simulink model "TP2"  (R2020a)
settings: Solver=VariableStepAuto  StartTime=0.0  StopTime=10.0  RelTol=1e-3
libraries: dspsigops x2, commutil2 x2, commrandsrc3 x1
settings Model: Creator=acer  LastModifiedBy=acer

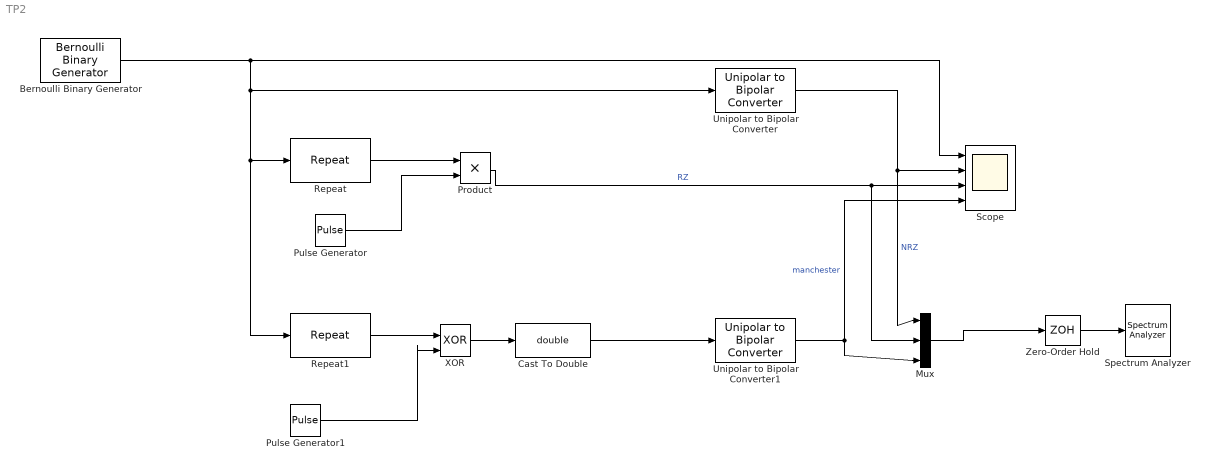
== system TP2 ==
  Bernoulli Binary Generator : commrandsrc3/Bernoulli Binary Generator  ProbabilityOfZero=0.5  SeedSource=Parameter  Seed=25  SampleTime=1  SamplesPerFrame=1  OutputDataType=double  SimulateUsing=Interpreted execution
  Cast To Double : DataTypeConversion  OutDataTypeStr=double
  Mux : Mux  Inputs=3
  Product : Product
  Pulse Generator : DiscretePulseGenerator  PulseType=Time based  Period=10  PulseWidth=5
  Pulse Generator1 : DiscretePulseGenerator  PulseType=Time based  Period=10  PulseWidth=5
  Repeat : dspsigops/Repeat  N=2  InputProcessing=Columns as channels (frame based)  RateOptions=Allow multirate processing  ic=0  mode=Unused parameter value
  Repeat1 : dspsigops/Repeat  N=2  InputProcessing=Columns as channels (frame based)  RateOptions=Allow multirate processing  ic=0  mode=Unused parameter value
  Scope : Scope  NumInputPorts=4
  Spectrum Analyzer : SpectrumAnalyzer  IsFrequencyInputMode=1
  Unipolar to Bipolar Converter : commutil2/Unipolar to Bipolar Converter  M=2  polarity=Positive  dataType=Inherit via internal rule
  Unipolar to Bipolar Converter1 : commutil2/Unipolar to Bipolar Converter  M=4  polarity=Positive  dataType=Inherit via internal rule
  XOR : Logic  Operator=XOR  IconShape=distinctive  AllPortsSameDT=off  OutDataTypeStr=boolean
  Zero-Order Hold : ZeroOrderHold  SampleTime=-1
  wires:
  Bernoulli Binary Generator/1 -> Unipolar to Bipolar Converter/1, Repeat1/1, Repeat/1, Scope/1
  Repeat/1 -> Product/1
  Pulse Generator/1 -> Product/2
  Product/1 -> Scope/3, Mux/2  "RZ"
  Unipolar to Bipolar Converter/1 -> Mux/1, Scope/2  "NRZ"
  Repeat1/1 -> XOR/1
  Pulse Generator1/1 -> XOR/2
  XOR/1 -> Cast To Double/1
  Cast To Double/1 -> Unipolar to Bipolar Converter1/1
  Unipolar to Bipolar Converter1/1 -> Scope/4, Mux/3  "manchester"
  Zero-Order Hold/1 -> Spectrum Analyzer/1
  Mux/1 -> Zero-Order Hold/1
